simulink model "JacobiTestbench"  (R2014b)
settings: Solver=ode45  StartTime=0.0  StopTime=10.0  RelTol=1e-3
settings Model: Creator=WKORMAX  LastModifiedBy=WKORMAX

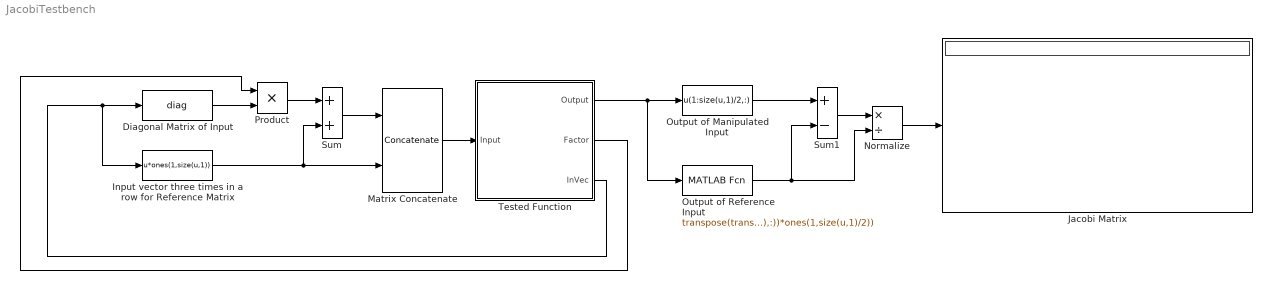
== system JacobiTestbench ==
  Diagonal Matrix of Input : MATLABFcn  MATLABFcn=diag  Output1D=off
  Input vector three times in a row for Reference Matrix : MATLABFcn  MATLABFcn=u*ones(1,size(u,1))  Output1D=off
  Jacobi Matrix : Display
  Matrix Concatenate : Concatenate  Mode=Multidimensional array  ConcatenateDimension=2
  Normalize : Product  Inputs=*/
  Output of Manipulated Input : MATLABFcn  MATLABFcn=u(1:size(u,1)/2,:)  Output1D=off
  Output of Reference Input : MATLABFcn  MATLABFcn=transpose(transpose(u(size(u,1):size(u,1),:))*ones(1,size(u,1)/2))  Output1D=off
  Product : Product
  Sum : Sum
  Sum1 : Sum  Inputs=+-
  Tested Function : Subsystem  Variant=on  VariantControl=Variant1  OverrideUsingVariant=Variant2
  wires:
  Input vector three times in a row for Reference Matrix/1 -> Matrix Concatenate/2, Sum/2
  Product/1 -> Sum/1
  Sum/1 -> Matrix Concatenate/1
  Tested Function/3(InVec) -> Input vector three times in a row for Reference Matrix/1, Diagonal Matrix of Input/1
  Output of Manipulated Input/1 -> Sum1/1
  Diagonal Matrix of Input/1 -> Product/2
  Output of Reference Input/1 -> Normalize/2, Sum1/2
  Sum1/1 -> Normalize/1
  Normalize/1 -> Jacobi Matrix/1
  Tested Function/2(Factor) -> Product/1
  Tested Function/1(Output) -> Output of Reference Input/1, Output of Manipulated Input/1
  Matrix Concatenate/1 -> Tested Function/1(Input)

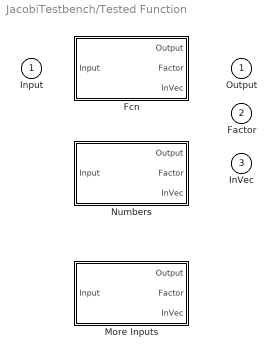
== system JacobiTestbench/Tested Function ==
  Input : Inport
  Fcn : Subsystem  VariantControl=Variant2
  More Inputs : Subsystem  VariantControl=Variant3
  Numbers : Subsystem  VariantControl=Variant1
  Output : Outport
  Factor : Outport  Port=2
  InVec : Outport  Port=3

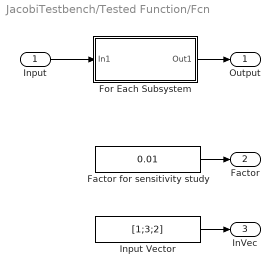
== system JacobiTestbench/Tested Function/Fcn ==
  Input : Inport
  Factor for sensitivity study : Constant  Value=0.01
  For Each Subsystem : Subsystem  TreatAsAtomicUnit=on
  Input Vector : Constant  Value=[1;3;2]
  Output : Outport
  Factor : Outport  Port=2
  InVec : Outport  Port=3
  wires:
  Input/1 -> For Each Subsystem/1(In1)
  For Each Subsystem/1(Out1) -> Output/1
  Factor for sensitivity study/1 -> Factor/1
  Input Vector/1 -> InVec/1

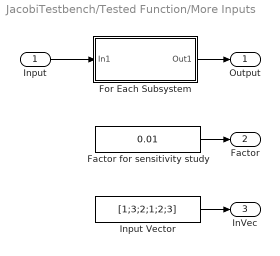
== system JacobiTestbench/Tested Function/More Inputs ==
  Input : Inport
  Factor for sensitivity study : Constant  Value=0.01
  For Each Subsystem : Subsystem  TreatAsAtomicUnit=on
  Input Vector : Constant  Value=[1;3;2;1;2;3]
  Output : Outport
  Factor : Outport  Port=2
  InVec : Outport  Port=3
  wires:
  Input/1 -> For Each Subsystem/1(In1)
  For Each Subsystem/1(Out1) -> Output/1
  Input Vector/1 -> InVec/1
  Factor for sensitivity study/1 -> Factor/1

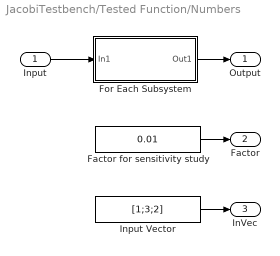
== system JacobiTestbench/Tested Function/Numbers ==
  Input : Inport
  Factor for sensitivity study : Constant  Value=0.01
  For Each Subsystem : Subsystem  TreatAsAtomicUnit=on
  Input Vector : Constant  Value=[1;3;2]
  Output : Outport
  Factor : Outport  Port=2
  InVec : Outport  Port=3
  wires:
  Input/1 -> For Each Subsystem/1(In1)
  For Each Subsystem/1(Out1) -> Output/1
  Input Vector/1 -> InVec/1
  Factor for sensitivity study/1 -> Factor/1

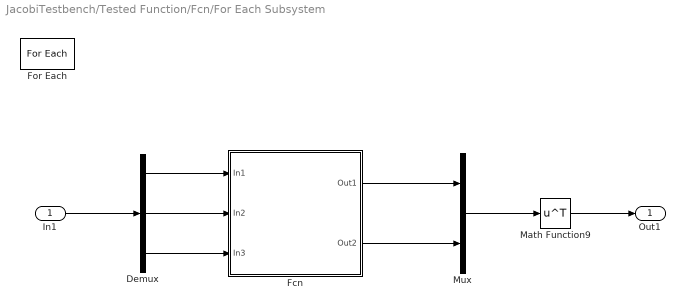
== system JacobiTestbench/Tested Function/Fcn/For Each Subsystem ==
  In1 : Inport  Partition=on  PartitionDimension=2  PartitionWidth=1
  Demux : Demux  Outputs=3
  Fcn : Subsystem  VariantControl=Variant1
  For Each : ForEach  DisableCoverage=on  IndexMode=One-based
  Math Function9 : Math  Operator=transpose  SaturateOnIntegerOverflow=on
  Mux : Mux  Inputs=2
  Out1 : Outport  ConcatenationDimension=1
  wires:
  Demux/2 -> Fcn/2(In2)
  Demux/1 -> Fcn/1(In1)
  Demux/3 -> Fcn/3(In3)
  In1/1 -> Demux/1
  Fcn/1(Out1) -> Mux/1
  Mux/1 -> Math Function9/1
  Fcn/2(Out2) -> Mux/2
  Math Function9/1 -> Out1/1

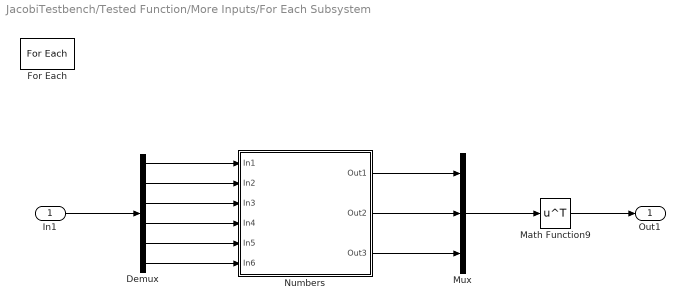
== system JacobiTestbench/Tested Function/More Inputs/For Each Subsystem ==
  In1 : Inport  Partition=on  PartitionDimension=2  PartitionWidth=1
  Demux : Demux  Outputs=6
  For Each : ForEach  DisableCoverage=on  IndexMode=One-based
  Math Function9 : Math  Operator=transpose  SaturateOnIntegerOverflow=on
  Mux : Mux  Inputs=3
  Numbers : Subsystem  VariantControl=Variant2
  Out1 : Outport  ConcatenationDimension=1
  wires:
  Demux/2 -> Numbers/2(In2)
  Demux/1 -> Numbers/1(In1)
  Demux/3 -> Numbers/3(In3)
  In1/1 -> Demux/1
  Numbers/1(Out1) -> Mux/1
  Mux/1 -> Math Function9/1
  Numbers/2(Out2) -> Mux/2
  Math Function9/1 -> Out1/1
  Demux/4 -> Numbers/4(In4)
  Demux/6 -> Numbers/6(In6)
  Demux/5 -> Numbers/5(In5)
  Numbers/3(Out3) -> Mux/3

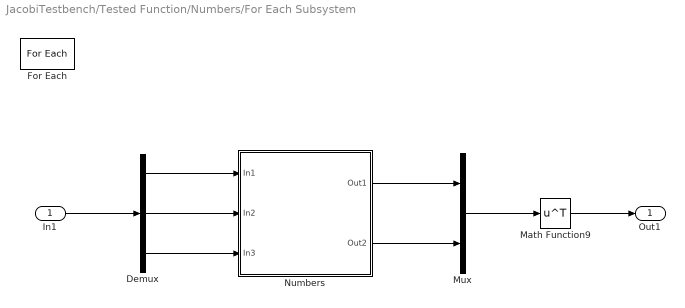
== system JacobiTestbench/Tested Function/Numbers/For Each Subsystem ==
  In1 : Inport  Partition=on  PartitionDimension=2  PartitionWidth=1
  Demux : Demux  Outputs=3
  For Each : ForEach  DisableCoverage=on  IndexMode=One-based
  Math Function9 : Math  Operator=transpose  SaturateOnIntegerOverflow=on
  Mux : Mux  Inputs=2
  Numbers : Subsystem  VariantControl=Variant2
  Out1 : Outport  ConcatenationDimension=1
  wires:
  Demux/2 -> Numbers/2(In2)
  Demux/1 -> Numbers/1(In1)
  Demux/3 -> Numbers/3(In3)
  In1/1 -> Demux/1
  Numbers/1(Out1) -> Mux/1
  Mux/1 -> Math Function9/1
  Numbers/2(Out2) -> Mux/2
  Math Function9/1 -> Out1/1

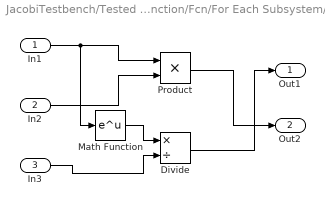
== system JacobiTestbench/Tested Function/Fcn/For Each Subsystem/Fcn ==
  In1 : Inport
  In2 : Inport  Port=2
  In3 : Inport  Port=3
  Divide : Product  Inputs=*/
  Math Function : Math  SaturateOnIntegerOverflow=on
  Product : Product
  Out1 : Outport
  Out2 : Outport  Port=2
  wires:
  In2/1 -> Product/2
  Product/1 -> Out2/1
  In1/1 -> Math Function/1, Product/1
  Math Function/1 -> Divide/1
  In3/1 -> Divide/2
  Divide/1 -> Out1/1

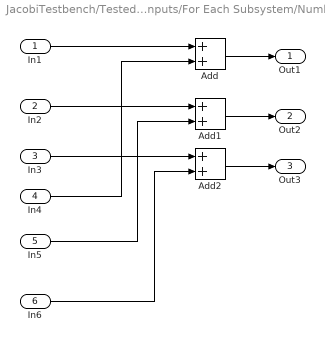
== system JacobiTestbench/Tested Function/More Inputs/For Each Subsystem/Numbers ==
  In1 : Inport
  In2 : Inport  Port=2
  In3 : Inport  Port=3
  In4 : Inport  Port=4
  In5 : Inport  Port=5
  In6 : Inport  Port=6
  Add : Sum
  Add1 : Sum
  Add2 : Sum
  Out1 : Outport
  Out2 : Outport  Port=2
  Out3 : Outport  Port=3
  wires:
  Add/1 -> Out1/1
  Add1/1 -> Out2/1
  In1/1 -> Add/1
  In2/1 -> Add1/1
  In3/1 -> Add2/1
  In4/1 -> Add/2
  In5/1 -> Add1/2
  In6/1 -> Add2/2
  Add2/1 -> Out3/1

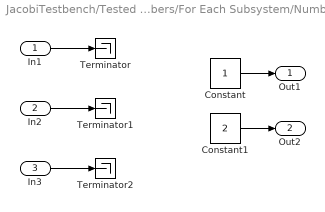
== system JacobiTestbench/Tested Function/Numbers/For Each Subsystem/Numbers ==
  In1 : Inport
  In2 : Inport  Port=2
  In3 : Inport  Port=3
  Constant : Constant
  Constant1 : Constant  Value=2
  Terminator : Terminator
  Terminator1 : Terminator
  Terminator2 : Terminator
  Out1 : Outport
  Out2 : Outport  Port=2
  wires:
  Constant1/1 -> Out2/1
  Constant/1 -> Out1/1
  In3/1 -> Terminator2/1
  In2/1 -> Terminator1/1
  In1/1 -> Terminator/1
